simulink model "M4_motor_load_gearbox_friction"  (Simulink 10.2)
settings: Solver=ode4  StartTime=0.0  StopTime=3  FixedStep=T_s*0.1  RelTol=1e-3
undefined symbols (not defined in the file): A_v, b_eq, b_v, J_eq, k, L, N_opt, omega_v, R, theta_0, V_bar
libraries: simulink x1
settings Model: Creator=ioannis  LastModifiedBy=mfocchi
settings DataIOCC: SaveFormat=Dataset  SignalLoggingSaveFormat=Dataset
settings OptimizationCC: LifeSpan=auto
settings DebuggingCC: UnderspecifiedInitializationDetection=Simplified  MergeDetectMultiDrivingBlocksExec=error  FcnCallInpInsideContextMsg=error  SFUnexpectedBacktrackingDiag=error  SFNoUnconditionalDefaultTransitionDiag=error  SFExecutionAtInitializationDiag=warning
settings HardwareCC: ProdBitPerPointer=64  ProdBitPerSizeT=64  ProdBitPerPtrDiffT=64  ProdLargestAtomicFloat=Float  ProdIntDivRoundTo=Zero  ProdEndianess=LittleEndian  ProdWordSize=64  ProdHWDeviceType=Intel->x86-64 (Windows64)
settings ModelReferenceCC: PropagateSignalLabelsOutOfModel=on
settings SFSimCC: SimUseLocalCustomCode=on
settings RTWCC: RTWUseLocalCustomCode=on
settings CodeAppCC: StateflowObjectComments=off
settings GRTTargetCC: TargetLangStandard=C99 (ISO)  CombineOutputUpdateFcns=on  GRTInterface=off
settings ConfigComp: CovMetricSettings=dwe  CovSaveCumulativeToWorkspaceVar=off  CovSaveSingleToWorkspaceVar=off  CovExternalEMLEnable=on

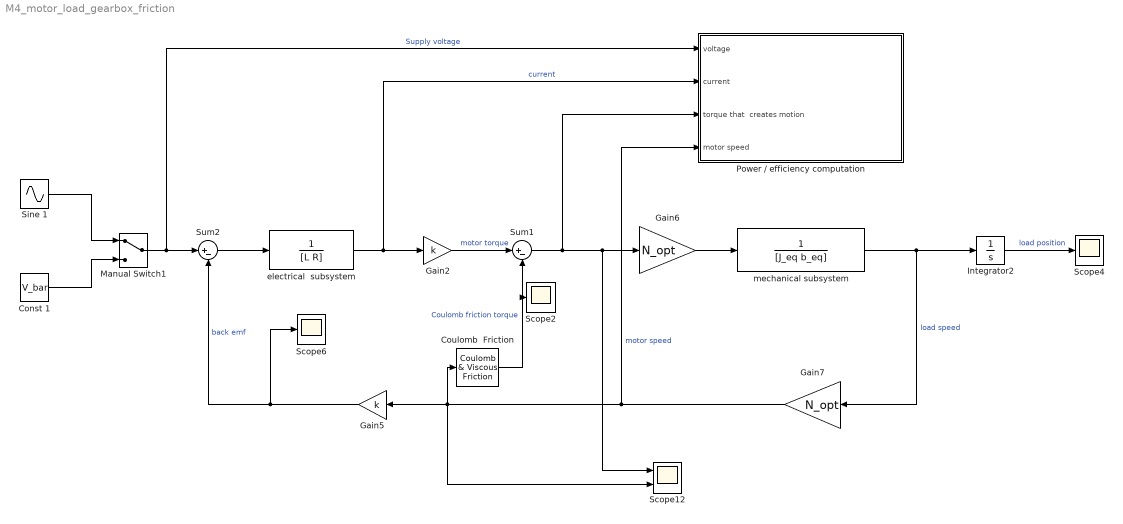
== system M4_motor_load_gearbox_friction ==
  Const 1 : Constant  Value=V_bar
  Coulomb  Friction : simulink/Discontinuities/Coulomb & Viscous Friction  offset=tau_c  gain=0
  Gain2 : Gain  Gain=k
  Gain5 : Gain  Gain=k
  Gain6 : Gain  Gain=N_opt
  Gain7 : Gain  Gain=N_opt
  Integrator2 : Integrator  InitialCondition=theta_0
  Manual Switch1 : ManualSwitch
  Power / efficiency computation : Subsystem
  Scope12 : Scope  NumInputPorts=2
  Scope2 : Scope
  Scope4 : Scope
  Scope6 : Scope
  Sine 1 : Sin  Amplitude=A_v  Bias=b_v  Frequency=omega_v  SampleTime=0
  Sum1 : Sum  Inputs=|+-
  Sum2 : Sum  Inputs=|+-
  electrical  subsystem : TransferFcn  Denominator=[L R]
  mechanical subsystem : TransferFcn  Denominator=[J_eq b_eq]
  wires:
  Gain7/1 -> Power / efficiency computation/4(motor speed), Scope12/2, Coulomb  Friction/1, Gain5/1  "motor speed"
  Manual Switch1/1 -> Power / efficiency computation/1(voltage), Sum2/1  "Supply voltage"
  Const 1/1 -> Manual Switch1/2
  mechanical subsystem/1 -> Gain7/1, Integrator2/1  "load speed"
  Gain5/1 -> Scope6/1, Sum2/2  "back emf"
  Sine 1/1 -> Manual Switch1/1
  Gain6/1 -> mechanical subsystem/1
  Integrator2/1 -> Scope4/1  "load position"
  Sum2/1 -> electrical  subsystem/1
  electrical  subsystem/1 -> Power / efficiency computation/2(current), Gain2/1  "current"
  Sum1/1 -> Power / efficiency computation/3(torque that  creates motion), Scope12/1, Gain6/1
  Gain2/1 -> Sum1/1  "motor torque"
  Coulomb  Friction/1 -> Scope2/1, Sum1/2  "Coulomb friction torque"

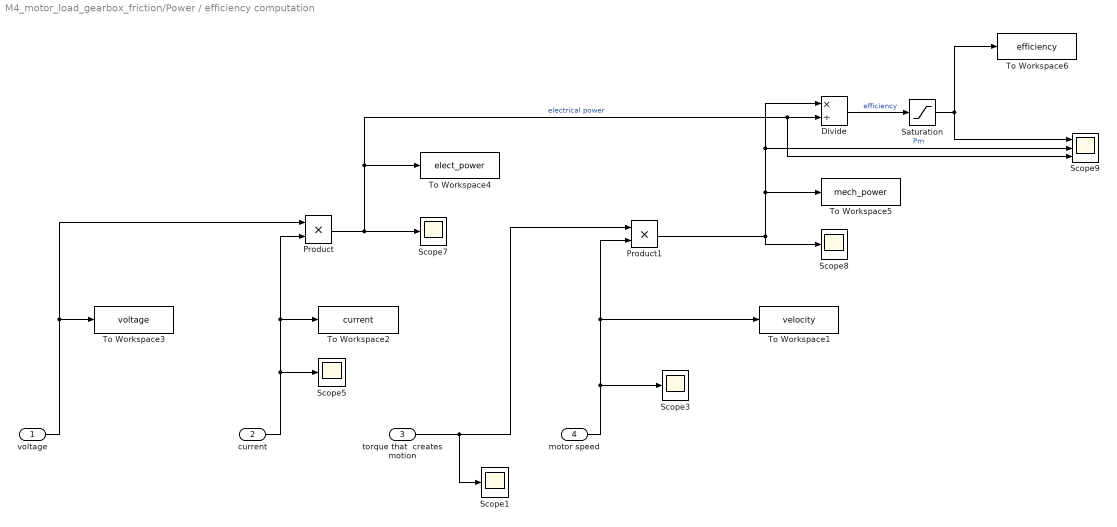
== system M4_motor_load_gearbox_friction/Power / efficiency computation ==
  voltage : Inport
  current : Inport  Port=2
  torque that  creates motion : Inport  Port=3
  motor speed : Inport  Port=4
  Divide : Product  Inputs=*/
  Product : Product
  Product1 : Product
  Saturation : Saturate  UpperLimit=1  LowerLimit=0
  Scope{1,3,5,7..8} (5 alike) : Scope
  Scope9 : Scope  NumInputPorts=3
  To Workspace1 : ToWorkspace  VariableName=velocity  SaveFormat=Timeseries  SampleTime=-1
  To Workspace2 : ToWorkspace  VariableName=current  SaveFormat=Timeseries  SampleTime=-1
  To Workspace3 : ToWorkspace  VariableName=voltage  SaveFormat=Timeseries  SampleTime=-1
  To Workspace4 : ToWorkspace  VariableName=elect_power  SaveFormat=Timeseries  SampleTime=-1
  To Workspace5 : ToWorkspace  VariableName=mech_power  SaveFormat=Timeseries  SampleTime=-1
  To Workspace6 : ToWorkspace  VariableName=efficiency  SaveFormat=Timeseries  SampleTime=-1
  wires:
  torque that  creates motion/1 -> Scope1/1, Product1/1
  motor speed/1 -> To Workspace1/1, Product1/2, Scope3/1
  voltage/1 -> Product/1, To Workspace3/1
  Product/1 -> Scope9/3, Divide/2, To Workspace4/1, Scope7/1  "electrical power"
  current/1 -> Product/2, To Workspace2/1, Scope5/1
  Divide/1 -> Saturation/1  "efficiency"
  Product1/1 -> Scope8/1, Divide/1, Scope9/2, To Workspace5/1  "Pm"
  Saturation/1 -> Scope9/1, To Workspace6/1
